simulink model "exemple_meca_emb_blocs_2"  (Simulink 8.1)
settings: Solver=ode45  StartTime=0.0  StopTime=20  RelTol=1e-3
values from neighbouring files (symbols this model uses):
  b_BV = 0.1    [init_modele_meca.m]
  b_M = 0.1    [init_modele_meca.m]
  I_BV = 0.1    [init_modele_meca.m]
  I_M = 0.2    [init_modele_meca.m]
  k = 0.5    [init_modele_meca.m]
  k_E = 0.5    [init_modele_meca.m]
settings Model: Creator=U243624  LastModifiedBy=U243624
settings DataIOCC: SignalLoggingSaveFormat=Dataset
settings OptimizationCC: ExpressionDepthLimit=128
settings DebuggingCC: FcnCallInpInsideContextMsg=EnableAllAsError
settings GRTTargetCC: CombineOutputUpdateFcns=on  GRTInterface=off

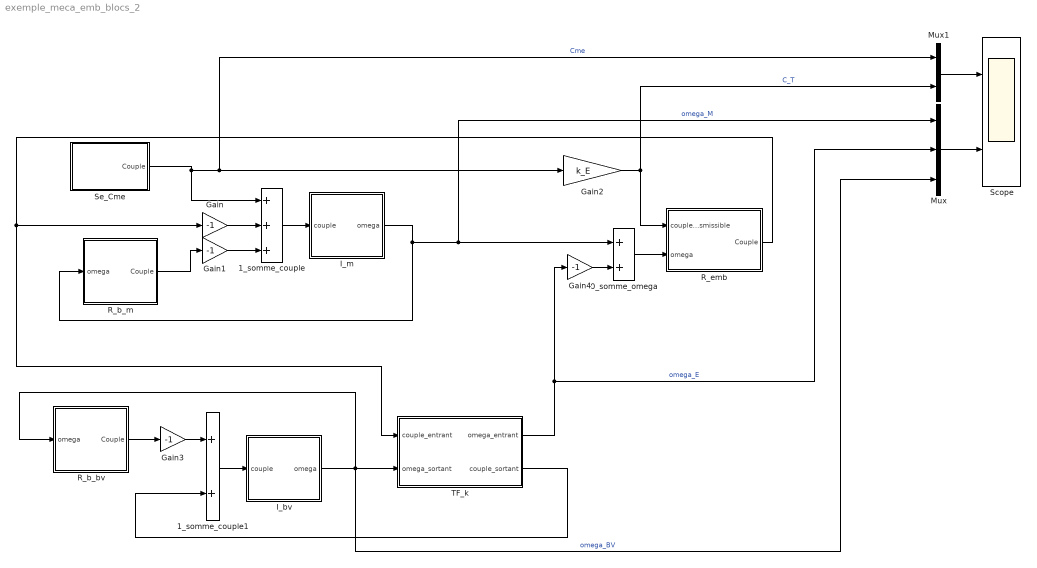
== system exemple_meca_emb_blocs_2 ==
  0_somme_omega : Sum
  1_somme_couple : Sum  Inputs=+++
  1_somme_couple1 : Sum
  Gain{,1,3..4} (4 alike) : Gain  Gain=-1
  Gain2 : Gain  Gain=k_E
  I_bv : Subsystem
  I_m : Subsystem
  Mux : Mux  Inputs=3
  Mux1 : Mux  Inputs=2
  R_b_bv : Subsystem
  R_b_m : Subsystem
  R_emb : Subsystem
  Scope : Scope  NumInputPorts=2
      settings: TimeRange=10  YMin=9.5~0  YMax=10.5~180
  Se_Cme : Subsystem
  TF_k : Subsystem
  wires:
  Se_Cme/1(Couple) -> Mux1/1, Gain2/1, 1_somme_couple/1  "Cme"
  R_b_m/1(Couple) -> Gain1/1
  R_emb/1(Couple) -> TF_k/1(couple_entrant), Gain/1
  1_somme_couple/1 -> I_m/1(couple)
  1_somme_couple1/1 -> I_bv/1(couple)
  R_b_bv/1(Couple) -> Gain3/1
  I_bv/1(omega) -> R_b_bv/1(omega), Mux/3, TF_k/2(omega_sortant)  "omega_BV"
  TF_k/1(omega_entrant) -> Mux/2, Gain4/1  "omega_E"
  I_m/1(omega) -> R_b_m/1(omega), Mux/1, 0_somme_omega/1  "omega_M"
  0_somme_omega/1 -> R_emb/2(omega)
  TF_k/2(couple_sortant) -> 1_somme_couple1/2
  Gain/1 -> 1_somme_couple/2
  Gain1/1 -> 1_somme_couple/3
  Gain2/1 -> Mux1/2, R_emb/1("couple_transmissible ")  "C_T"
  Gain3/1 -> 1_somme_couple1/1
  Gain4/1 -> 0_somme_omega/2
  Mux/1 -> Scope/2
  Mux1/1 -> Scope/1

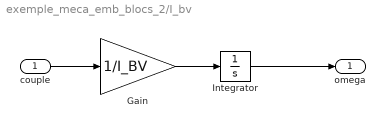
== system exemple_meca_emb_blocs_2/I_bv ==
  couple : Inport
  Gain : Gain  Gain=1/I_BV
  Integrator : Integrator
  omega : Outport
  wires:
  couple/1 -> Gain/1
  Integrator/1 -> omega/1
  Gain/1 -> Integrator/1

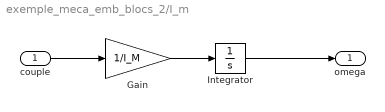
== system exemple_meca_emb_blocs_2/I_m ==
  couple : Inport
  Gain : Gain  Gain=1/I_M
  Integrator : Integrator
  omega : Outport
  wires:
  couple/1 -> Gain/1
  Integrator/1 -> omega/1
  Gain/1 -> Integrator/1

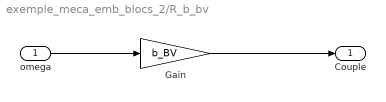
== system exemple_meca_emb_blocs_2/R_b_bv ==
  omega : Inport
  Gain : Gain  Gain=b_BV
  Couple : Outport
  wires:
  omega/1 -> Gain/1
  Gain/1 -> Couple/1

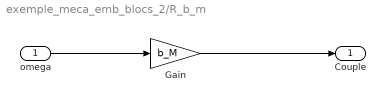
== system exemple_meca_emb_blocs_2/R_b_m ==
  omega : Inport
  Gain : Gain  Gain=b_M
  Couple : Outport
  wires:
  omega/1 -> Gain/1
  Gain/1 -> Couple/1

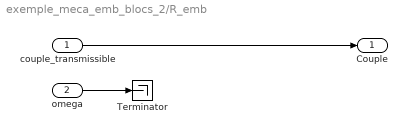
== system exemple_meca_emb_blocs_2/R_emb ==
  "couple_transmissible " : Inport
  omega : Inport  Port=2
  Terminator : Terminator
  Couple : Outport
  wires:
  omega/1 -> Terminator/1
  "couple_transmissible "/1 -> Couple/1

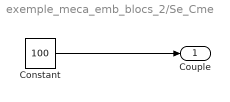
== system exemple_meca_emb_blocs_2/Se_Cme ==
  Constant : Constant  Value=100
  Couple : Outport
  wires:
  Constant/1 -> Couple/1

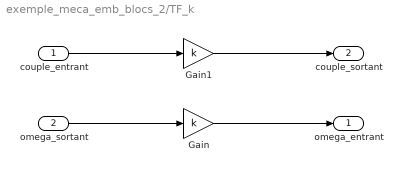
== system exemple_meca_emb_blocs_2/TF_k ==
  couple_entrant : Inport
  omega_sortant : Inport  Port=2
  Gain : Gain  Gain=k
  Gain1 : Gain  Gain=k
  omega_entrant : Outport
  couple_sortant : Outport  Port=2
  wires:
  omega_sortant/1 -> Gain/1
  couple_entrant/1 -> Gain1/1
  Gain/1 -> omega_entrant/1
  Gain1/1 -> couple_sortant/1
